simulink model "controller_velocity_input_shaping_lqr"  (R2021a)
settings: Solver=FixedStepAuto  StartTime=0.0  StopTime=10.0  RelTol=1e-3
undefined symbols (not defined in the file): control_angles, Dnotch_disc_DENOM, Dnotch_disc_NUM, EKF_freq, freq_factor, g, hover_init, K_notch, l, max_tilt, max_total_T, max_vel_xy, mp, mq, Q_lqr, R_lqr, sim_freq, thr_max, thr_min, type, zeta_p_notch, zeta_z_notch
libraries: simulink x1, dspswit3 x1, powerlib_meascontrol x1
settings Model: Creator=francois  LastModifiedBy=esl
settings SolverCC: AlgebraicLoopSolver=TrustRegion
settings DebuggingCC: SFMachineParentedDataDiag=warning
settings ModelReferenceCC: ModelReferenceNumInstancesAllowed=Single

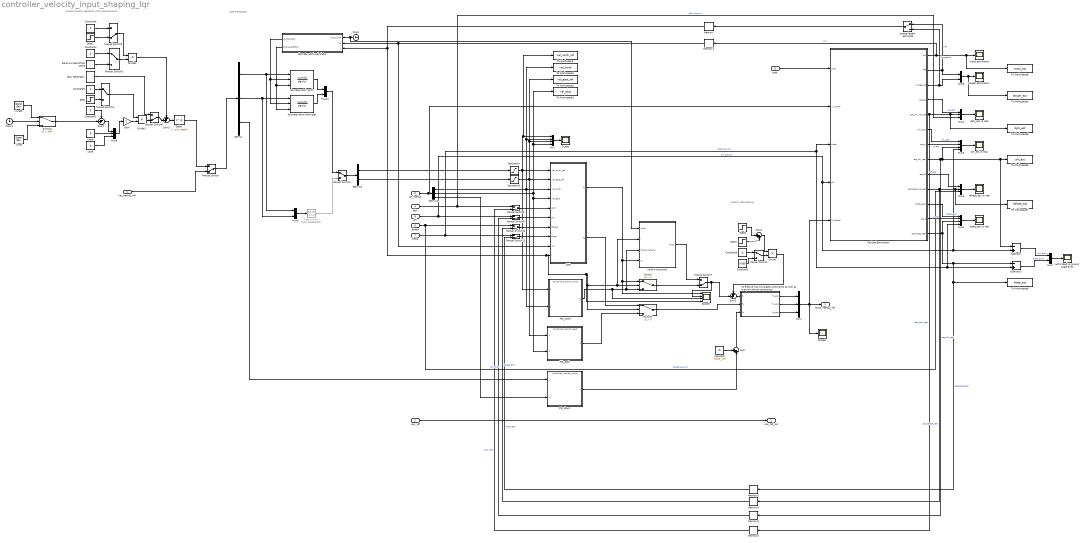
== system controller_velocity_input_shaping_lqr ==
  note: velocity disturbance
  note: manual velocity setpoints with noise and such
  note: INPUT SHAPING
  "vel_inertial_ref " : Inport  PortDimensions=3
  yaw_ref : Inport  Port=2
  vel_inertial : Inport  Port=3
  dphi : Inport  Port=4
  phi : Inport  Port=5
  dtheta : Inport  Port=6
  theta : Inport  Port=7
  quat : Inport  Port=8
  Band-Limited White Noise : simulink/Sources/Band-Limited White Noise  Cov=1e-2  Ts=100/sim_freq  seed=[23341]
  Clock : Clock
  Clock1 : Clock
  Constant : Constant  Value=-hover_init
  Constant1 : Constant  Value=0
  Constant2 : Constant  Value=0.005
  Constant3 : Constant  Value=0
  Constant4 : Constant  Value=0
  Constant5 : Constant
  Constant6 : Constant
  Delay : Delay  DelayLength=sim_freq*0
  Demux : Demux  Outputs=3
  Demux1 : Demux  Outputs=3
  Demux2 : Demux  Outputs=2
  Divide : Product  Inputs=**
  Divide1 : Product  Inputs=**
  Divide2 : Product  Inputs=**
  Gain : Gain  Gain=-1
  LQR : Subsystem
  Manual Switch{,5..11} (8 alike) : ManualSwitch  CurrentSetting=0
  Manual Switch{1..4} (4 alike) : ManualSwitch
  Memory{,1..5} (6 alike) : Memory
  Mux : Mux
  Mux{1,4..5,8} (4 alike) : Mux  Inputs=3
  Mux{6..7,9..10} (4 alike) : Mux  Inputs=2
  Mux2 : Mux
  Mux3 : Mux
  PID_down : ModelReference  ModelNameDialog=controller_velocity_down.slx  SimulationMode=Normal  ModelReferenceVersion=3.4
  "PID_east " : ModelReference  ModelNameDialog=controller_velocity_east.slx  SimulationMode=Normal  ModelReferenceVersion=3.3
  PID_north : ModelReference  ModelNameDialog=controller_velocity_north.slx  SimulationMode=Normal  ModelReferenceVersion=3.4
  Payload Estimation : Subsystem
  "Rate Limiter " : RateLimiter  Commented=on  RisingSlewLimit=25/(2*pi*4.67)  FallingSlewLimit=-25/(2*pi*4.67)  SampleTimeMode=inherited
  Saturation : Saturate  UpperLimit=max_vel_xy  LowerLimit=-max_vel_xy
  Saturation1 : Saturate  UpperLimit=max_vel_xy  LowerLimit=-max_vel_xy
  Scope : Scope
  Scope1 : Scope  NumInputPorts=4
  Scope2 : Scope
  Stair Generator : powerlib_meascontrol/Pulse & Signal Generators/Stair Generator  t=10*[0, 1, 2, 3, 4, 5, 6, 7, 8, 9, 10]  e=-[0, 1, 2, 3, 4, 5, 6, 7, 8, 9, 10]  Ts=1/sim_freq
  Step : Step  Time=100  Before=1  After=12  SampleTime=0
  Step1 : Step  Time=175  SampleTime=0
  Step2 : Step  Time=40  SampleTime=0
  Step3 : Step  Time=10000  SampleTime=0
  Subtract : Sum  Inputs=-+
  Subtract1 : Sum  Inputs=-+
  Sum : Sum  Inputs=++|
  Sum1 : Sum  Inputs=-+|
  Sum2 : Sum  Inputs=++|
  Sum3 : Sum  Inputs=++|
  Sum4 : Sum  Inputs=|++
  Switch : Switch  Criteria=u2 > Threshold
  Switch1 : Switch  Criteria=u2 > Threshold
  Switch2 : Switch  Criteria=u2 > Threshold  Threshold=400
  To Workspace : ToWorkspace  VariableName=vel_north_ref  SampleTime=-1
  To Workspace1 : ToWorkspace  VariableName=vel_north  SampleTime=-1
  To Workspace2 : ToWorkspace  VariableName=vel_east_ref  SampleTime=-1
  To Workspace3 : ToWorkspace  VariableName=vel_east  SampleTime=-1
  To Workspace4 : ToWorkspace  VariableName=length_est  SampleTime=-1
  To Workspace5 : ToWorkspace  VariableName=dphi_est  SampleTime=-1
  To Workspace6 : ToWorkspace  VariableName=phi_est  SampleTime=-1
  To Workspace7 : ToWorkspace  VariableName=dtheta_est  SampleTime=-1
  To Workspace8 : ToWorkspace  VariableName=theta_est  SampleTime=-1
  To Workspace9 : ToWorkspace  VariableName=mass_est  SampleTime=-1
  To enforce max tilt angles constraints as well as max/min thrust constraints : MATLAB Function  TreatAsAtomicUnit=on  SystemSampleTime=1/sim_freq
  Veref : Constant  Value=0
  Vnref : SignalGenerator  WaveForm=square  Amplitude=1/2*1  Frequency=1/(40*1)
  Vnref1 : SignalGenerator  WaveForm=square  Amplitude=1/2*24  Frequency=1/(40*4)
  choose length estimate : ManualSwitch
  "control transition " : MATLAB Function  TreatAsAtomicUnit=on
  discrete notch north : DiscreteTransferFcn  NumeratorSource=Input port  Numerator=Dnotch_disc_NUM  DenominatorSource=Input port  Denominator=Dnotch_disc_DENOM  a0EqualsOne=on
      settings: InputPortMap=u0,p1,p3
  discrete notch north east : DiscreteTransferFcn  NumeratorSource=Input port  Numerator=Dnotch_disc_NUM  DenominatorSource=Input port  Denominator=Dnotch_disc_DENOM  a0EqualsOne=on
      settings: InputPortMap=u0,p1,p3
  discrete notch calculator : MATLAB Function  TreatAsAtomicUnit=on
  dphi_est vs real : Scope
  dtheta_est vs real : Scope
  estimated vs ground angle error : Scope
  length estimation : Scope
  mass estimation : Scope
  phi_est vs real : Scope
  theta_est vs real : Scope
  vdref : Constant  Value=0
  force_inertial_ref : Outport
  yaw_ref_out : Outport  Port=2
  wires:
  Payload Estimation/4(est_dp) -> Mux4/1  "dp_est"
  Demux/3 -> PID_down/1
  vel_inertial/1 -> Demux1/1, Payload Estimation/2(v_inertial)
  choose length estimate/1 -> Memory/1
  Memory1/1 -> LQR/9(mp), discrete notch calculator/2(mp)
  Mux1/1 -> Payload Estimation/5(F_inertial), force_inertial_ref/1, Scope2/1
  Payload Estimation/3(l bisgaardt) -> Mux6/2, choose length estimate/2  "l bisgaardt"
  Constant/1 -> Sum/1
  Payload Estimation/12(est_t) -> Mux2/2  "t_est"
  Payload Estimation/10(est_theta_vel_real) -> Memory4/1, To Workspace7/1, Mux5/2  "est_dtheta_real"
  dtheta/1 -> Mux5/3, Manual Switch10/1  "dtheta ground"
  To enforce max tilt angles constraints as well as max/min thrust constraints/2(fy_sat) -> Mux1/2
  LQR/1(fn) -> Scope1/1, Switch/1, "control transition "/4(fn)
  Demux1/3 -> PID_down/2
  Sum/1 -> To enforce max tilt angles constraints as well as max/min thrust constraints/3(fz)
  Mux/1 -> Scope/1
  theta/1 -> Manual Switch11/1, Payload Estimation/3(theta), Mux2/4, Subtract1/2  "theta ground"
  phi/1 -> Manual Switch9/1, Subtract/2, Mux3/4, Payload Estimation/4("phi ")  "phi ground"
  Payload Estimation/6(phi_cam) -> Mux3/1  "phi_cam"
  LQR/2(fe) -> Switch1/1
  Payload Estimation/11(theta_cam) -> Mux2/1  "theta_cam"
  Payload Estimation/13(est_theta_real) -> Mux2/3, Subtract1/1, Memory5/1, To Workspace8/1  "est_theta_real"
  Memory/1 -> Scope1/4, Switch1/2, "control transition "/2(l), Switch/2, LQR/10(l), discrete notch calculator/3(l)
  Demux1/2 -> "PID_east "/2, LQR/4("vel_east "), Mux/4, To Workspace3/1
  Subtract1/1 -> Mux7/2  "theta error"
  Switch1/1 -> To enforce max tilt angles constraints as well as max/min thrust constraints/2(fy)
  Payload Estimation/1(mp) -> To Workspace9/1, mass estimation/1, Memory1/1  "mp"
  Payload Estimation/7(est_p) -> Mux3/2  "p_est"
  PID_down/1 -> Sum/2
  Payload Estimation/5(est_phi_vel_real) -> To Workspace5/1, Mux4/2, Memory2/1  "est_dphi_real"
  To enforce max tilt angles constraints as well as max/min thrust constraints/1(fx_sat) -> Mux1/1
  Mux3/1 -> phi_est vs real/1
  quat/1 -> Payload Estimation/1(quat)
  dphi/1 -> Mux4/3, Manual Switch8/1  "dphi ground"
  Subtract/1 -> Mux7/1  "phi error"
  "PID_east "/1 -> Switch1/3
  Mux5/1 -> dtheta_est vs real/1
  Mux7/1 -> estimated vs ground angle error/1
  Payload Estimation/8(est_phi_real) -> To Workspace6/1, Subtract/1, Mux3/3, Memory3/1  "est_phi_real"
  PID_north/1 -> Scope1/3, "control transition "/3(force_inertial_n), Switch/3
  Payload Estimation/9(est_dt) -> Mux5/1  "dt_est"
  yaw_ref/1 -> yaw_ref_out/1
  Payload Estimation/2("l fft ") -> Mux6/1, choose length estimate/1  "l fft"
  Mux6/1 -> length estimation/1, To Workspace4/1
  To enforce max tilt angles constraints as well as max/min thrust constraints/3(fz_sat) -> Mux1/3
  Saturation1/1 -> LQR/2(vel_east_ref), "PID_east "/1, Mux/3, To Workspace2/1
  Mux4/1 -> dphi_est vs real/1
  Saturation/1 -> LQR/1(vel_north_ref), PID_north/1, To Workspace/1, Mux/1
  Demux/1 -> Mux9/1, discrete notch north/1
  Demux/2 -> Mux9/2, discrete notch north east/1
  discrete notch calculator/1(D_disc_NUM) -> discrete notch north east/2, discrete notch north/2
  discrete notch calculator/2(D_disc_DENOM) -> discrete notch north east/3, discrete notch north/3
  Clock/1 -> "control transition "/1(clock), discrete notch calculator/1(clock_time)
  Memory2/1 -> Manual Switch8/2  "dphi EKF"
  Memory3/1 -> Manual Switch9/2  "phi EKF"
  Memory4/1 -> Manual Switch10/2  "dtheta EKF"
  Memory5/1 -> Manual Switch11/2  "theta EKF"
  Manual Switch5/1 -> Divide2/1
  Divide2/1 -> Sum3/1
  Sum3/1 -> Delay/1
  Manual Switch3/1 -> Divide2/2
  Divide1/1 -> Manual Switch6/2
  Constant1/1 -> Sum1/1
  Stair Generator/1 -> Manual Switch6/1
  Step2/1 -> Manual Switch5/2
  Constant4/1 -> Manual Switch3/1
  Manual Switch4/1 -> Divide1/1
  Constant6/1 -> Manual Switch5/1
  Manual Switch6/1 -> Sum3/2
  Constant5/1 -> Manual Switch4/1
  Gain/1 -> Divide1/2
  Band-Limited White Noise/1 -> Manual Switch3/2
  Step/1 -> Manual Switch4/2
  Constant3/1 -> Manual Switch2/1
  Manual Switch2/1 -> Divide/2
  Divide/1 -> Sum2/1
  Step1/1 -> Sum4/2
  Constant2/1 -> Manual Switch2/2
  Sum2/1 -> To enforce max tilt angles constraints as well as max/min thrust constraints/1(fx)
  "vel_inertial_ref "/1 -> Manual Switch/2
  Manual Switch/1 -> Demux/1
  Sum1/1 -> Mux8/1
  Veref/1 -> Mux8/2
  vdref/1 -> Mux8/3
  Mux8/1 -> Gain/1
  Delay/1 -> Manual Switch/1
  Mux2/1 -> theta_est vs real/1
  Manual Switch1/1 -> Demux2/1
  Demux2/1 -> Saturation/1
  Demux2/2 -> Saturation1/1
  Mux9/1 -> "Rate Limiter "/1
  "Rate Limiter "/1 -> Manual Switch1/2
  discrete notch north/1 -> Mux10/1
  discrete notch north east/1 -> Mux10/2
  Mux10/1 -> Manual Switch1/1
  Demux1/1 -> PID_north/2, LQR/3(vel_north), To Workspace1/1, Mux/2
  "control transition "/1(force) -> Manual Switch7/1
  Switch/1 -> Manual Switch7/2
  Manual Switch7/1 -> Scope1/2, Sum2/2
  Manual Switch8/1 -> LQR/5(dphi)
  Manual Switch9/1 -> LQR/6("phi ")
  Manual Switch10/1 -> LQR/7(dtheta)
  Manual Switch11/1 -> LQR/8(theta)
  Step3/1 -> Sum4/1
  Sum4/1 -> Divide/1
  Vnref/1 -> Switch2/3
  Switch2/1 -> Sum1/2
  Vnref1/1 -> Switch2/1
  Clock1/1 -> Switch2/2

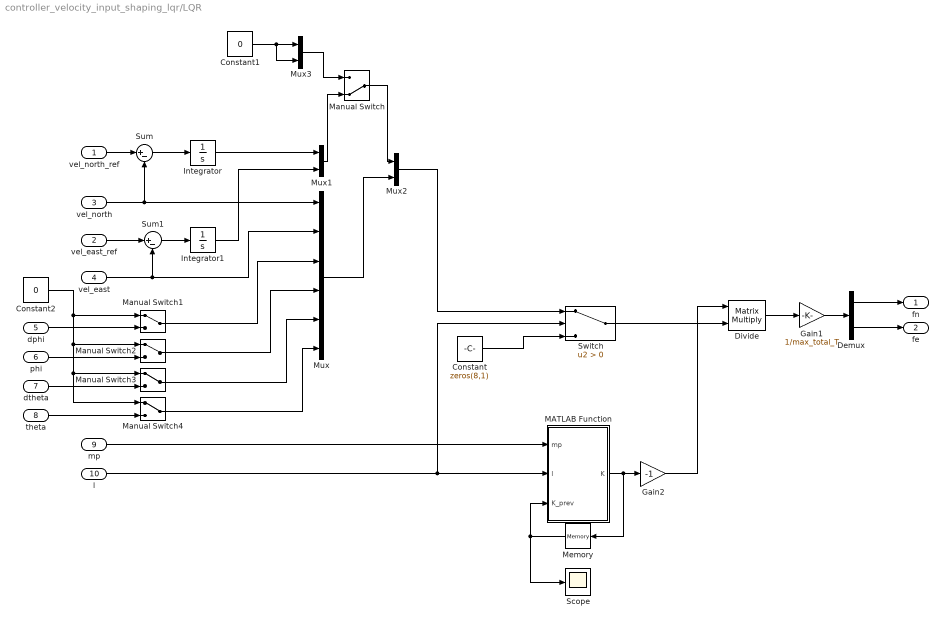
== system controller_velocity_input_shaping_lqr/LQR ==
  vel_north_ref : Inport
  vel_east_ref : Inport  Port=2
  vel_north : Inport  Port=3
  "vel_east " : Inport  Port=4
  dphi : Inport  Port=5
  "phi " : Inport  Port=6
  dtheta : Inport  Port=7
  theta : Inport  Port=8
  mp : Inport  Port=9
  l : Inport  Port=10
  Constant : Constant  Value=zeros(8,1)
  Constant1 : Constant  Value=0
  Constant2 : Constant  Value=0
  Demux : Demux  Outputs=2
  Divide : Product  Inputs=**  Multiplication=Matrix(*)
  Gain1 : Gain  Gain=1/max_total_T
  Gain2 : Gain  Gain=-1
  Integrator : Integrator
  Integrator1 : Integrator
  MATLAB Function : MATLAB Function  TreatAsAtomicUnit=on
  Manual Switch : ManualSwitch  CurrentSetting=0
  Manual Switch{1..4} (4 alike) : ManualSwitch
  Memory : Memory
  Mux : Mux  Inputs=6
  Mux1 : Mux  Inputs=2
  Mux2 : Mux  Inputs=2
  Mux3 : Mux  Inputs=2
  Scope : Scope
  Sum : Sum  Inputs=|+-
  Sum1 : Sum  Inputs=|+-
  Switch : Switch  Criteria=u2 > Threshold
  fn : Outport  VectorParamsAs1DForOutWhenUnconnected=off
  fe : Outport  Port=2  VectorParamsAs1DForOutWhenUnconnected=off
  wires:
  vel_north_ref/1 -> Sum/1
  vel_north/1 -> Sum/2, Mux/1
  Mux2/1 -> Switch/1
  Constant/1 -> Switch/3
  MATLAB Function/1(K) -> Memory/1, Gain2/1
  mp/1 -> MATLAB Function/1(mp)
  l/1 -> Switch/2, MATLAB Function/2(l)
  Divide/1 -> Gain1/1
  Switch/1 -> Divide/2
  Gain2/1 -> Divide/1
  Memory/1 -> MATLAB Function/3(K_prev), Scope/1
  vel_east_ref/1 -> Sum1/1
  Sum1/1 -> Integrator1/1
  "vel_east "/1 -> Sum1/2, Mux/2
  Integrator1/1 -> Mux1/2
  Sum/1 -> Integrator/1
  Integrator/1 -> Mux1/1
  Mux/1 -> Mux2/2
  Gain1/1 -> Demux/1
  Demux/1 -> fn/1
  Demux/2 -> fe/1
  Manual Switch/1 -> Mux2/1
  Mux1/1 -> Manual Switch/2
  Mux3/1 -> Manual Switch/1
  Constant1/1 -> Mux3/2, Mux3/1
  Constant2/1 -> Manual Switch4/1, Manual Switch3/1, Manual Switch2/1, Manual Switch1/1
  dphi/1 -> Manual Switch1/2
  Manual Switch1/1 -> Mux/3
  "phi "/1 -> Manual Switch2/2
  dtheta/1 -> Manual Switch3/2
  Manual Switch2/1 -> Mux/4
  Manual Switch3/1 -> Mux/5
  Manual Switch4/1 -> Mux/6
  theta/1 -> Manual Switch4/2

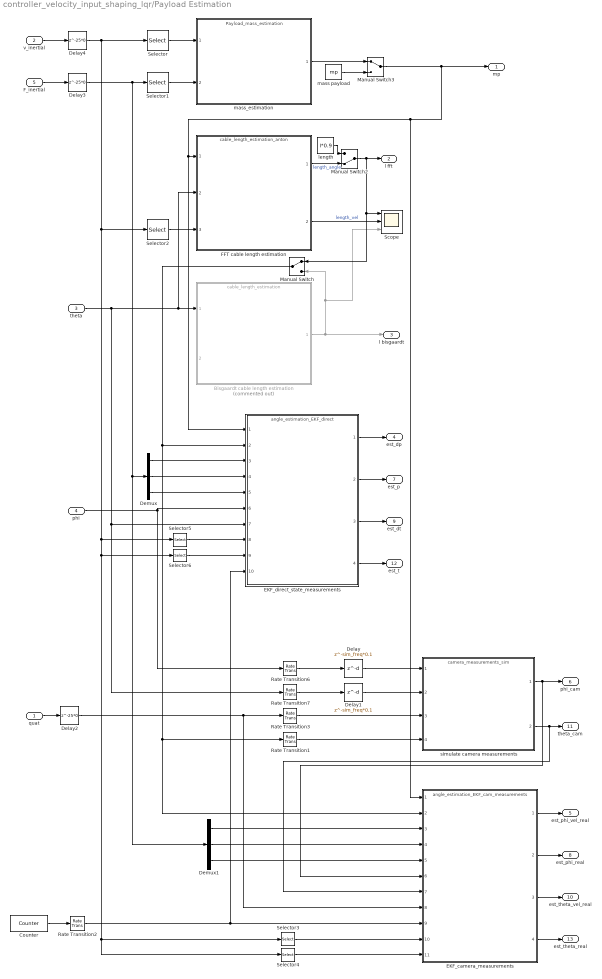
== system controller_velocity_input_shaping_lqr/Payload Estimation ==
  quat : Inport  PortDimensions=4  SampleTime=1/sim_freq
  v_inertial : Inport  Port=2  SampleTime=1/sim_freq
  theta : Inport  Port=3
  "phi " : Inport  Port=4  SampleTime=1/sim_freq
  F_inertial : Inport  Port=5
  Bisgaardt cable length estimation : ModelReference  Commented=on  ModelNameDialog=cable_length_estimation.slx  SimulationMode=Normal  ModelReferenceVersion=1.52
  Counter : dspswit3/Counter  Direction=Up  CountEvent=Free running  CounterSize=User defined  MaxCount=sim_freq/EKF_freq  InitialCount=1  Output=Count  HitValue=10  ResetInput=off  SamplesPerFrame=1  Ts=1/sim_freq  CntDtype=double  HitDtype=Logical
  Delay : Delay  DelayLength=sim_freq*0.1
  Delay1 : Delay  DelayLength=sim_freq*0.1
  Delay2 : Delay  DelayLength=25*0
  Delay3 : Delay  DelayLength=25*0
  Delay4 : Delay  DelayLength=25*0
  Demux : Demux  Outputs=3
  Demux1 : Demux  Outputs=3
  EKF_camera_measurements : ModelReference  ModelNameDialog=angle_estimation_EKF_cam_measurements.slx  SimulationMode=Normal  ModelReferenceVersion=1.132
  EKF_direct_state_measurements : ModelReference  ModelNameDialog=angle_estimation_EKF_direct.slx  SimulationMode=Normal  ModelReferenceVersion=1.28
  FFT cable length estimation : ModelReference  ModelNameDialog=cable_length_estimation_anton.slx  SimulationMode=Normal  ModelReferenceVersion=1.13
  Manual Switch : ManualSwitch
  Manual Switch2 : ManualSwitch  CurrentSetting=0
  Manual Switch3 : ManualSwitch
  Rate Transition{1..3,6..7} (5 alike) : RateTransition  OutPortSampleTime=1/(sim_freq)
  Scope : Scope  NumInputPorts=3
  Selector : Selector  InputPortWidth=3  IndexOptions=Index vector (dialog)  Indices=3  OutputSizes=1
  Selector1 : Selector  InputPortWidth=3  IndexOptions=Index vector (dialog)  Indices=3  OutputSizes=1
  Selector2 : Selector  InputPortWidth=3  IndexOptions=Index vector (dialog)  Indices=1  OutputSizes=1
  Selector3 : Selector  InputPortWidth=3  IndexOptions=Index vector (dialog)  Indices=1  OutputSizes=1
  Selector4 : Selector  InputPortWidth=3  IndexOptions=Index vector (dialog)  Indices=2  OutputSizes=1
  Selector5 : Selector  InputPortWidth=3  IndexOptions=Index vector (dialog)  Indices=1  OutputSizes=1
  Selector6 : Selector  InputPortWidth=3  IndexOptions=Index vector (dialog)  Indices=2  OutputSizes=1
  length : Constant  Value=l*0.9
  mass payload : Constant  Value=mp
  "mass_estimation " : ModelReference  ModelNameDialog=Payload_mass_estimation.slx  SimulationMode=Normal  ModelReferenceVersion=1.33
  simulate camera measurements : ModelReference  ModelNameDialog=camera_measurements_sim.slx  SimulationMode=Normal  ModelReferenceVersion=1.56
  mp : Outport  SampleTime=1/sim_freq
  "l fft " : Outport  Port=2
  l bisgaardt : Outport  Port=3
  est_dp : Outport  Port=4
  est_phi_vel_real : Outport  Port=5
  phi_cam : Outport  Port=6
  est_p : Outport  Port=7
  est_phi_real : Outport  Port=8
  est_dt : Outport  Port=9
  est_theta_vel_real : Outport  Port=10
  theta_cam : Outport  Port=11
  est_t : Outport  Port=12
  est_theta_real : Outport  Port=13
  wires:
  v_inertial/1 -> Delay4/1
  Selector/1 -> "mass_estimation "/1
  Selector1/1 -> "mass_estimation "/2
  FFT cable length estimation/1 -> Manual Switch2/2  "length_angle"
  Bisgaardt cable length estimation/1 -> Scope/3, Manual Switch/2, l bisgaardt/1
  theta/1 -> FFT cable length estimation/2, Bisgaardt cable length estimation/1, Rate Transition7/1, EKF_direct_state_measurements/7
  "phi "/1 -> EKF_direct_state_measurements/6, Rate Transition6/1
  Demux/1 -> EKF_direct_state_measurements/3
  Demux/2 -> EKF_direct_state_measurements/4
  Demux/3 -> EKF_direct_state_measurements/5
  EKF_direct_state_measurements/1 -> est_dp/1
  EKF_direct_state_measurements/2 -> est_p/1
  EKF_direct_state_measurements/3 -> est_dt/1
  EKF_direct_state_measurements/4 -> est_t/1
  FFT cable length estimation/2 -> Scope/2  "length_vel"
  Selector2/1 -> FFT cable length estimation/3
  Demux1/1 -> EKF_camera_measurements/3
  Demux1/2 -> EKF_camera_measurements/4
  Demux1/3 -> EKF_camera_measurements/5
  EKF_camera_measurements/1 -> est_phi_vel_real/1
  EKF_camera_measurements/2 -> est_phi_real/1
  EKF_camera_measurements/3 -> est_theta_vel_real/1
  EKF_camera_measurements/4 -> est_theta_real/1
  Counter/1 -> Rate Transition2/1
  quat/1 -> Delay2/1
  F_inertial/1 -> Delay3/1
  simulate camera measurements/1 -> EKF_camera_measurements/6, phi_cam/1
  simulate camera measurements/2 -> EKF_camera_measurements/7, theta_cam/1
  Rate Transition6/1 -> Delay/1
  Rate Transition7/1 -> Delay1/1
  "mass_estimation "/1 -> Manual Switch3/1
  Rate Transition1/1 -> simulate camera measurements/4
  Rate Transition3/1 -> simulate camera measurements/3
  Rate Transition2/1 -> EKF_camera_measurements/9, EKF_direct_state_measurements/10
  Manual Switch/1 -> Rate Transition1/1, EKF_camera_measurements/2, EKF_direct_state_measurements/2
  Delay/1 -> simulate camera measurements/1
  Delay1/1 -> simulate camera measurements/2
  Selector3/1 -> EKF_camera_measurements/10
  Selector4/1 -> EKF_camera_measurements/11
  Manual Switch2/1 -> "l fft "/1, Manual Switch/1, Scope/1
  length/1 -> Manual Switch2/1
  mass payload/1 -> Manual Switch3/2
  Manual Switch3/1 -> EKF_camera_measurements/1, EKF_direct_state_measurements/1, FFT cable length estimation/1, mp/1
  Delay2/1 -> Rate Transition3/1, EKF_camera_measurements/8
  Delay3/1 -> Demux1/1, Demux/1, Selector1/1
  Delay4/1 -> Selector/1, Selector3/1, Selector4/1, Selector6/1, Selector5/1, Selector2/1
  Selector5/1 -> EKF_direct_state_measurements/8
  Selector6/1 -> EKF_direct_state_measurements/9

== matlab function controller_velocity_input_shaping_lqr/To enforce max tilt angles constraints as well as max//min thrust constraints ==
  data: fx input; fx_sat output; fy input; fz input; fy_sat output; max_tilt parameter; thr_max parameter; fz_sat output; thr_min parameter
function [fx_sat, fy_sat, fz_sat] = constrain_max_tilt(fx, fy, fz, max_tilt, thr_max, thr_min)
    % First constrain fz.
    if fz > -thr_min
        fz_sat = -thr_min;
    elseif fz < -thr_max
        fz_sat = -thr_max;
    else
        fz_sat = fz;
    end
    
    % Constrain fx and fy
    thrust_max_NE_tilt = abs(fz_sat) * tan(max_tilt * pi/180);
    thrust_max_NE = sqrt(thr_max*thr_max - fz_sat*fz_sat);
    thrust_max_NE = min(thrust_max_NE_tilt, thrust_max_NE);
    
    fx_sat = fx;
    fy_sat = fy;

%     if dot([fx, fy], [fx, fy]) > thrust_max_NE*thrust_max_NE
%         mag = norm([fx, fy]);
    mag = norm([fx, fy]); %myne
    if mag > thrust_max_NE% myne
        fx_sat = fx / mag * thrust_max_NE;
        fy_sat = fy / mag * thrust_max_NE;
    end
end

== matlab function controller_velocity_input_shaping_lqr/LQR/MATLAB Function ==
  data: mp input; K output; l input; K_prev input; mq parameter; g parameter; max_total_T parameter; Q_lqr parameter; R_lqr parameter; sim_freq parameter; control_angles parameter
function K = lqr_gain(mp, l, K_prev, mq, g, max_total_T, Q_lqr, R_lqr, sim_freq, control_angles)
    % states = [dVn, dVe, Vn, Ve, dphi, phi, dtheta, theta]

    coder.extrinsic('lqr');
    coder.extrinsic('lqrd');
    
    K = zeros(2,8);
    if l > 0 
        if all(K_prev) == 0

                    % dVn,      dVe,         Vn,        Ve,         dphi,       phi,        dtheta,     theta]
            Ass_aug= [0          0           -1         0           0           0           0           0;
                      0          0           0          -1          0           0           0           0;
                      0          0           0          0           0           0           0           (mp/mq)*g;
                      0          0           0          0           0       (g*mp)/mq       0           0;
                      0          0           0          0           0   -g*(mq+mp)/(l*mq)   0           0;
                      0          0           0          0           1           0           0           0;
                      0          0           0          0           0           0           0           -g*(mq+mp)/(l*mq);
                      0          0           0          0           0           0           1           0];

            
            Bss_aug = [0        0;
                   0        0;
                 1/mq       0;
                   0       1/mq;
                   0    -1/(l*mq);
                   0        0;
               -1/(l*mq)    0;
                 0          0];             


                           %*2     *2
            %Q_lqr = diag([50*0.5 50*0.5 50*1 50*1 2/100 3/100 2/100 3/100]); %50 50 /100 /100 /100
            %R_lqr = 3*diag([1 1]); %3 %%5 met 100 werk ook goed
            %%Q_lqr = diag([1/(15^2) 1/(15^2) 1/(12^2) 1/(12^2) 2/((180*2*pi)^2) 3/((180*2*pi)^2) 2/((180*2*pi)^2) 3/((180*2*pi)^2)]);
            %%R_lqr = diag([1/(max_total_T^2) 1/(max_total_T^2)]);

            K = lqr(Ass_aug, Bss_aug, Q_lqr, R_lqr);
            %K = lqrd(Ass_aug, Bss_aug, Q_lqr, R_lqr, 1/sim_freq);
            
            if control_angles == 0
                K(1, 8) = 0;
                K(2, 6) = 0;
            end

            
        else
            K = K_prev;
        end
    end

end

== matlab function controller_velocity_input_shaping_lqr/discrete notch calculator ==
  data: clock_time input; mp input; l input; D_disc_NUM output; D_disc_DENOM output; zeta_z_notch parameter; zeta_p_notch parameter; mq parameter; sim_freq parameter; K_notch parameter; type parameter; freq_factor parameter
function [D_disc_NUM, D_disc_DENOM]  = notch_filter(clock_time, mp, l, zeta_z_notch, zeta_p_notch, mq, sim_freq, K_notch, type, freq_factor)
D_disc_NUM = zeros(1, 3);
D_disc_DENOM = zeros(1, 3); 
ohm = 0;

C = 0;
D = 0;
b0 = 0;
b1 = 0;
b2 = 0;
a1 = 0;
a2 = 0;
coder.extrinsic('tf');
coder.extrinsic('c2d');
coder.extrinsic('tfdata');


if l > 0% && clock_time >= 200  

    if type == 1
        %% notch filter 
        ohm = sqrt((9.81*(mp+mq))/(l*mq))*freq_factor;% 1.1 0.85 1.0
        
        Dnotch = K_notch*tf([1/ohm^2 2*zeta_z_notch/ohm 1], [1/ohm^2 2*zeta_p_notch/ohm 1]);
        Dnotch_discrete = c2d(Dnotch, 1/sim_freq);
        [D_disc_NUM, D_disc_DENOM] = tfdata(Dnotch_discrete, 'v');
       

    else
        % moet dalk anton se manier hier gebruik
       %% LPF
       ohm = sqrt((9.81*(mp+mq))/(l*mq))*0.8; %0.6
       Dlpf = K_notch*tf([ohm^2], [1 2*sqrt(2)*ohm ohm^2]);
       Dlpf_discrete = c2d(Dlpf, 1/sim_freq);
       [D_disc_NUM, D_disc_DENOM] = tfdata(Dlpf_discrete, 'v');
    end
else
    D_disc_NUM = [1 1 1];
    D_disc_DENOM = [1 1 1]; 
    ohm = 0;
end


end

== matlab function controller_velocity_input_shaping_lqr/control transition  ==
  data: clock input; l input; force output; force_inertial_n input; fn input
function force  = control_transition(clock, l, force_inertial_n, fn)
force = 0;


if l>0
    if clock > 70
        force = fn;
    else
        force = force_inertial_n;
    end
else
    force = force_inertial_n;
end
